simulink model "pipt1_flt"  (R2017b)
settings: Solver=ode1  StartTime=0.0  StopTime=0.1  FixedStep=0.0001  RelTol=1e-3  AbsTol=1e-6
settings Model: Tag=0  ExtModeTrigMode=oneshot  ExtModeArmWhenConnect=off  Creator=dSPACE GmbH  LastModifiedBy=dSPACE GmbH
settings DataIOCC: SaveFormat=Array
settings OptimizationCC: BlockReduction=off  BooleanDataType=off  OptimizeBlockIOStorage=off  BufferReuse=off  GlobalBufferReuse=off  ExpressionFolding=off  ExpressionDepthLimit=2147483647  LocalBlockOutputs=off  InitFltsAndDblsToZero=on  LifeSpan=inf
settings DebuggingCC: SaveWithParameterizedLinksMsg=none  UnderspecifiedInitializationDetection=Classic  MergeDetectMultiDrivingBlocksExec=none  SignalResolutionControl=TryResolveAllWithWarning  MultiTaskDSMMsg=warning  MultiTaskCondExecSysMsg=none  FcnCallInpInsideContextMsg=warning  BusObjectLabelMismatch=error  StateNameClashWarn=warning  StrictBusMsg=ErrorOnBusTreatedAsVector  NonBusSignalsTreatedAsBus=error  SFUnexpectedBacktrackingDiag=warning  SFNoUnconditionalDefaultTransitionDiag=warning  SFExecutionAtInitializationDiag=none
settings HardwareCC: ProdBitPerPointer=32  ProdBitPerSizeT=32  ProdBitPerPtrDiffT=32  ProdLargestAtomicFloat=None  ProdIntDivRoundTo=Undefined  ProdEndianess=Unspecified  ProdWordSize=32  ProdHWDeviceType=32-bit Generic  TargetUnknown=on
settings ModelReferenceCC: PropagateSignalLabelsOutOfModel=off
settings RTWCC: TemplateMakefile=grt_vc.tmf
settings CodeAppCC: StateflowObjectComments=on
settings GRTTargetCC: TargetFcnLib=ansi_tfl_tmw.mat  TargetLangStandard=C89/C90 (ANSI)  ModelReferenceCompliant=off  GeneratePreprocessorConditionals=Disable all  CombineOutputUpdateFcns=off  MatFileLogging=off  GRTInterface=on
settings ConfigComp: CovMetricSettings=dw  CovHtmlReporting=on  CovSaveCumulativeToWorkspaceVar=on  CovSaveSingleToWorkspaceVar=on  CovExternalEMLEnable=off

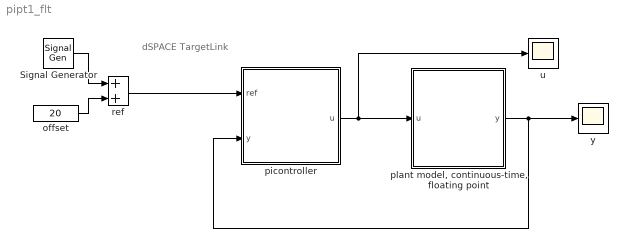
== system pipt1_flt ==
  note: dSPACE TargetLink
  Signal Generator : SignalGenerator  WaveForm=square  Amplitude=5  Frequency=20
  offset : Constant  Value=20
  picontroller : Subsystem
  "plant model, continuous-time, floating point" : Subsystem
  ref : Sum  SaturateOnIntegerOverflow=on  InputSameDT=on  OutDataTypeStr=Inherit: Same as first input
  u : Scope
  y : Scope
  wires:
  ref/1 -> picontroller/1(ref)
  Signal Generator/1 -> ref/1
  offset/1 -> ref/2
  picontroller/1(u) -> "plant model, continuous-time, floating point"/1(u), u/1
  "plant model, continuous-time, floating point"/1(y) -> picontroller/2(y), y/1

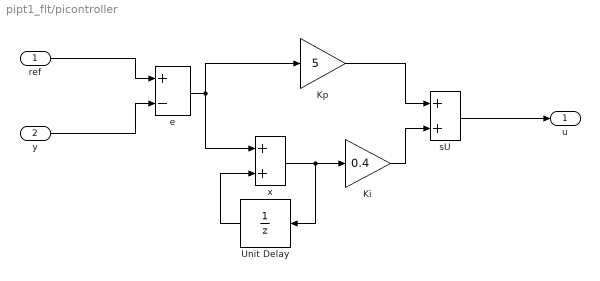
== system pipt1_flt/picontroller ==
  ref : Inport  PortDimensions=1  SampleTime=1e-4
  y : Inport  Port=2  PortDimensions=1  SampleTime=1e-4
  Ki : Gain  Gain=0.4  SaturateOnIntegerOverflow=on  OutDataTypeStr=Inherit: Same as input  ParamDataTypeStr=Inherit: Same as input
  Kp : Gain  Gain=5  SaturateOnIntegerOverflow=on  OutDataTypeStr=Inherit: Same as input  ParamDataTypeStr=Inherit: Same as input
  Unit Delay : UnitDelay  SampleTime=0.0001
  e : Sum  Inputs=+-  SaturateOnIntegerOverflow=on  InputSameDT=on  OutDataTypeStr=Inherit: Same as first input
  sU : Sum  SaturateOnIntegerOverflow=on  InputSameDT=on  OutDataTypeStr=Inherit: Same as first input
  x : Sum  SaturateOnIntegerOverflow=on  InputSameDT=on  OutDataTypeStr=Inherit: Same as first input
  u : Outport  InitialOutput=0
  wires:
  Ki/1 -> sU/2
  e/1 -> x/1, Kp/1
  Kp/1 -> sU/1
  x/1 -> Ki/1, Unit Delay/1
  Unit Delay/1 -> x/2
  ref/1 -> e/1
  y/1 -> e/2
  sU/1 -> u/1

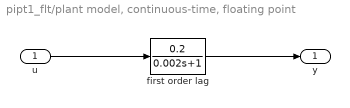
== system pipt1_flt/plant model, continuous-time, floating point ==
  u : Inport
  first order lag : TransferFcn  Numerator=[0.2]  Denominator=[0.002 1]
  y : Outport  InitialOutput=0
  wires:
  u/1 -> first order lag/1
  first order lag/1 -> y/1
